simulink model "Prop_VV_2"  (R2020b)
settings: Solver=VariableStepAuto  StartTime=0.0  StopTime=10.0  RelTol=1e-3
settings Model: Creator=Jonathan van Zyl  LastModifiedBy=Jonathan van Zyl

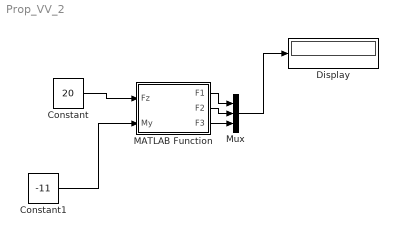
== system Prop_VV_2 ==
  Constant : Constant  Value=20
  Constant1 : Constant  Value=-11
  Display : Display
  MATLAB Function : MATLAB Function  TreatAsAtomicUnit=on
  Mux : Mux  Inputs=3
  wires:
  Constant1/1 -> MATLAB Function/2(My)
  Constant/1 -> MATLAB Function/1(Fz)
  MATLAB Function/1(F1) -> Mux/1
  MATLAB Function/2(F2) -> Mux/2
  MATLAB Function/3(F3) -> Mux/3
  Mux/1 -> Display/1

== matlab function Prop_VV_2/MATLAB Function ==
  data: Fz input; F1 output; My input; F2 output; F3 output
function [F1, F2, F3] = func(Fz, My)
a = 1.2598;
b = 2.2598;
c = -1.3402;

F = Fz;
M = My;
syms x y z
eq1 = 2*x+2*y+4*z==F;
eq2 = 2*a*x+2*b*y+4*c*z==M;

xyz = solve([eq1, eq2]);
x = xyz.x
x_fun = matlabFunction(x);

y = xyz.y
y_fun = matlabFunction(y);

syms t
func = sqrt(x_fun(t)^2+y_fun(t)^2+t^2);

test = matlabFunction(func);

result = fminbnd(test,-10000,10000);

F1 = x_fun(result);
F2 = y_fun(result);
F3 = result;

total = sqrt(F1^2 + F2^2 + F3^2);
end
